simulink library "marlo_lib_v01"  (Simulink 8.1)
settings: Solver=ode45  StartTime=0.0  StopTime=10.0  RelTol=1e-3
undefined symbols (not defined in the file or in its folder): A_deriv_encoder, A_deriv_IMU, ANOMALY_INIT, B_deriv_encoder, B_deriv_IMU, C_deriv_encoder, C_deriv_IMU, CalibrationParams, Com1, D_deriv_encoder, D_deriv_IMU, Dt_deriv_encoder, Dt_deriv_IMU, EncoderAngleLimits, EncoderThreshold, IMUAngleLimits, IMUParams, IMUThreshold, KVHOrientationCal, m_XR17D15x, MAX_ANOMALY, MotorParams, none, standard, x0_deriv_encoder, x0_deriv_IMU, XOFF, XON
libraries: xpcethercatlib x307, speedgoatlib x26, xpcseriallib x15, simulink x8, marlo_lib_v01 x6, dspswit3 x2, xpclib x1
(part 1 of 6)
settings Model: Creator=bgbuss  LastModifiedBy=bgbuss

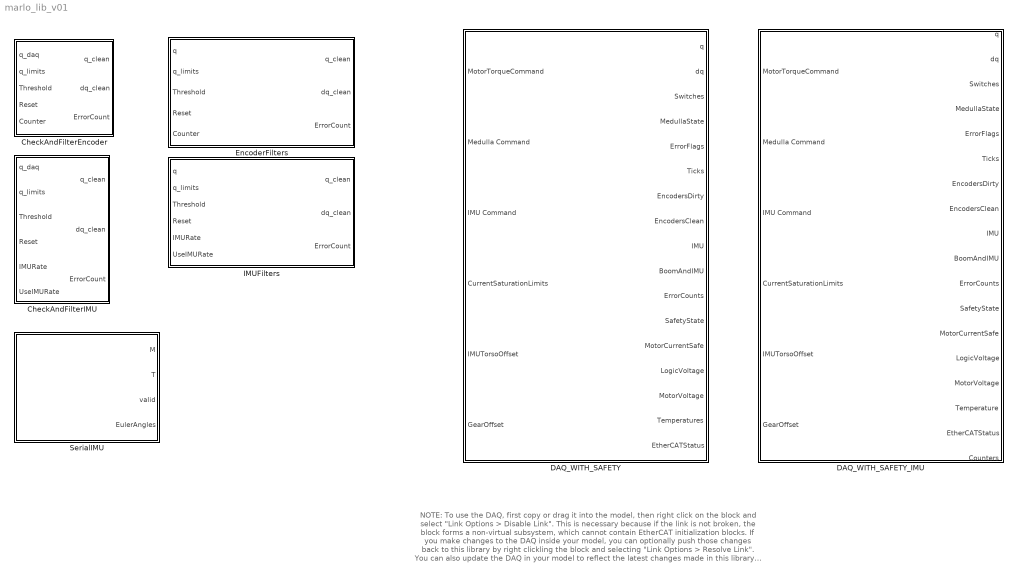
== system marlo_lib_v01 ==
  note: NOTE: To use the DAQ, first copy or drag it into the model,
      | then right click on the block and select "Link Options > Disable Link".
      | This is necessary because if the link is not broken, the block forms a
      | non-virtual subsystem, which cannot contain EtherCAT initialization blocks.
      |
      | If you make changes to the DAQ inside your model, you can optionally push
      | those changes back to this library by right clickling the block and selecting
      | "Link Options > Resolve Link". You can also update the DAQ in your model
      | to reflect the latest changes made in this library by selecting "Link Options >
      | Resolve Link" and pulling (RESTORE) the changes into your model.
  CheckAndFilterEncoder : Subsystem
  CheckAndFilterIMU : Subsystem
  DAQ_WITH_SAFETY : Subsystem
  DAQ_WITH_SAFETY_IMU : Subsystem  AncestorBlock=marlo_lib_v01/DAQ_WITH_SAFETY
  EncoderFilters : Subsystem  TreatAsAtomicUnit=on
  IMUFilters : Subsystem  TreatAsAtomicUnit=on
  SerialIMU : Subsystem

== system marlo_lib_v01/CheckAndFilterEncoder ==
  q_daq : Inport
  q_limits : Inport  Port=2
  Threshold : Inport  Port=3
  Reset : Inport  Port=4
  Counter : Inport  Port=5
  AnomalyDetection : Stateflow chart  TreatAsAtomicUnit=on  SystemSampleTime=Dt_deriv_encoder
  Constant : Constant  Value=Dt_deriv_encoder
  Discrete State-Space : DiscreteStateSpace  A=A_deriv_encoder  B=B_deriv_encoder  C=C_deriv_encoder  D=D_deriv_encoder  X0=x0_deriv_encoder  SampleTime=Dt_deriv_encoder
  Unit Delay : UnitDelay  SampleTime=Dt_deriv_encoder
  q_clean : Outport
  dq_clean : Outport  Port=2
  ErrorCount : Outport  Port=3
  wires:
  AnomalyDetection/1(q_clean) -> Discrete State-Space/1, q_clean/1
  Discrete State-Space/1 -> dq_clean/1, Unit Delay/1
  q_daq/1 -> AnomalyDetection/1(q)
  Threshold/1 -> AnomalyDetection/5(Threshold)
  Unit Delay/1 -> AnomalyDetection/2(dq)
  Constant/1 -> AnomalyDetection/7(ANOMALY_DT)
  q_limits/1 -> AnomalyDetection/4(q_limits)
  AnomalyDetection/2(ErrorCount) -> ErrorCount/1
  Reset/1 -> AnomalyDetection/6(Reset)
  Counter/1 -> AnomalyDetection/3(Counter)

== system marlo_lib_v01/CheckAndFilterIMU ==
  q_daq : Inport
  q_limits : Inport  Port=2
  Threshold : Inport  Port=3
  Reset : Inport  Port=4
  IMURate : Inport  Port=5
  UseIMURate : Inport  Port=6
  AnomalyDetection : Stateflow chart  TreatAsAtomicUnit=on  SystemSampleTime=Dt_deriv_IMU
  Constant : Constant  Value=Dt_deriv_IMU
  Discrete State-Space : DiscreteStateSpace  A=A_deriv_IMU  B=B_deriv_IMU  C=C_deriv_IMU  D=D_deriv_IMU  X0=x0_deriv_IMU  SampleTime=Dt_deriv_IMU
  Rate Transition{,3..7} (6 alike) : RateTransition  OutPortSampleTimeMultiple=2
  Rate Transition1 : RateTransition  Deterministic=off  OutPortSampleTime=.001
  Rate Transition2 : RateTransition  Deterministic=off  OutPortSampleTime=.001
  Rate Transition8 : RateTransition  Deterministic=off  OutPortSampleTime=.001
  Switch : Switch  Criteria=u2 ~= 0  Threshold=0.5
  Unit Delay : UnitDelay  SampleTime=Dt_deriv_IMU
  q_clean : Outport
  dq_clean : Outport  Port=2
  ErrorCount : Outport  Port=3
  wires:
  Unit Delay/1 -> AnomalyDetection/2(dq)
  Threshold/1 -> Rate Transition5/1
  q_daq/1 -> Rate Transition/1
  AnomalyDetection/1(q_clean) -> Discrete State-Space/1, Rate Transition1/1
  Rate Transition/1 -> AnomalyDetection/1(q)
  Rate Transition1/1 -> q_clean/1
  Rate Transition2/1 -> dq_clean/1
  Switch/1 -> Rate Transition2/1, Unit Delay/1
  Discrete State-Space/1 -> Switch/3
  IMURate/1 -> Rate Transition3/1
  UseIMURate/1 -> Rate Transition4/1
  Constant/1 -> AnomalyDetection/6(ANOMALY_DT)
  Rate Transition3/1 -> Switch/1
  Rate Transition4/1 -> Switch/2
  Rate Transition5/1 -> AnomalyDetection/4(Threshold)
  q_limits/1 -> Rate Transition6/1
  Reset/1 -> Rate Transition7/1
  Rate Transition6/1 -> AnomalyDetection/3(q_limits)
  Rate Transition7/1 -> AnomalyDetection/5(Reset)
  AnomalyDetection/2(ErrorCount) -> Rate Transition8/1
  Rate Transition8/1 -> ErrorCount/1

== system marlo_lib_v01/DAQ_WITH_SAFETY ==
  MotorTorqueCommand : Inport
  Medulla Command : Inport  Port=2
  IMU Command : Inport  Port=3
  CurrentSaturationLimits : Inport  Port=4
  IMUTorsoOffset : Inport  Port=5
  GearOffset : Inport  Port=6
  DAQ : Subsystem
  Data Type Conversion15 : DataTypeConversion  OutDataTypeStr=double
  Gain : Gain  Gain=-1
  SAFETY : MATLAB Function  TreatAsAtomicUnit=on
  Saturation Dynamic : simulink/Discontinuities/Saturation Dynamic  OutMin=[]  OutMax=[]  OutDataTypeStr=Inherit: Same as second input  OutDataType=fixdt(1, 16)  OutScaling=2^-10  DoSatur=off
  Terminator2 : Terminator
  Terminator5 : Terminator
  TorqueToCurrent : Gain  Gain=[10; 10; 5.5; 10; 10; 5.5]
  Unit Delay : UnitDelay  SampleTime=-1
  q : Outport
  dq : Outport  Port=2
  Switches : Outport  Port=3
  MedullaState : Outport  Port=4
  ErrorFlags : Outport  Port=5
  Ticks : Outport  Port=6
  EncodersDirty : Outport  Port=7
  EncodersClean : Outport  Port=8
  IMU : Outport  Port=9
  BoomAndIMU : Outport  Port=10
  ErrorCounts : Outport  Port=11
  SafetyState : Outport  Port=12
  MotorCurrentSafe : Outport  Port=13
  LogicVoltage : Outport  Port=14
  MotorVoltage : Outport  Port=15
  Temperatures : Outport  Port=16
  EtherCATStatus : Outport  Port=17
  wires:
  DAQ/17(EtherCATStatus) -> EtherCATStatus/1
  DAQ/4(ToeSwitches) -> Terminator2/1
  DAQ/12(EncodersDirty) -> EncodersDirty/1
  DAQ/11(Ticks) -> Ticks/1
  SAFETY/3(IMUCommandSafe) -> DAQ/3(IMU Command)
  MotorTorqueCommand/1 -> TorqueToCurrent/1
  Medulla Command/1 -> SAFETY/2(MedullaCommand)
  IMU Command/1 -> SAFETY/3(IMUCommand)
  DAQ/1(q) -> SAFETY/4(q), q/1
  DAQ/2(dq) -> SAFETY/5(dq), dq/1
  DAQ/3(LimitSwitches) -> SAFETY/6(Switches), Switches/1
  DAQ/8(LogicVoltage) -> LogicVoltage/1, SAFETY/8(LogicVoltage)
  DAQ/14(IMU) -> IMU/1
  SAFETY/4(SafetyStateOut) -> SafetyState/1
  TorqueToCurrent/1 -> Saturation Dynamic/2  "current_unsat"
  DAQ/10(Thermistors) -> Temperatures/1, SAFETY/7(Thermistors)
  DAQ/7(MotorVoltage) -> MotorVoltage/1
  DAQ/9(AmpMeasuredCurrent) -> Terminator5/1
  DAQ/5(MedullaState) -> MedullaState/1
  DAQ/6(ErrorFlags) -> ErrorFlags/1
  Saturation Dynamic/1 -> Data Type Conversion15/1
  CurrentSaturationLimits/1 -> Saturation Dynamic/1, Gain/1
  Gain/1 -> Saturation Dynamic/3
  SAFETY/1(MotorCurrentCommandSafe) -> DAQ/1(Motor Command), MotorCurrentSafe/1
  SAFETY/2(MedullaCommandSafe) -> DAQ/2(Medulla Command)
  Data Type Conversion15/1 -> SAFETY/1(MotorCurrentCommand)  "current_sat"
  DAQ/15(BoomAndIMU) -> BoomAndIMU/1
  IMUTorsoOffset/1 -> DAQ/4(IMUTorsoOffset)
  GearOffset/1 -> DAQ/5(GearOffset)
  SAFETY/5(SafetyCountOut) -> Unit Delay/1
  Unit Delay/1 -> SAFETY/9(SafetyCountIn)
  DAQ/16(ErrorCounts) -> ErrorCounts/1
  DAQ/13(EncodersClean) -> EncodersClean/1

== system marlo_lib_v01/DAQ_WITH_SAFETY_IMU ==
  MotorTorqueCommand : Inport
  Medulla Command : Inport  Port=2
  IMU Command : Inport  Port=3
  CurrentSaturationLimits : Inport  Port=4
  IMUTorsoOffset : Inport  Port=5
  GearOffset : Inport  Port=6
  DAQ : Subsystem
  Data Type Conversion15 : DataTypeConversion  OutDataTypeStr=double
  Gain : Gain  Gain=-1
  SAFETY : MATLAB Function  TreatAsAtomicUnit=on
  Saturation Dynamic : simulink/Discontinuities/Saturation Dynamic  OutMin=[]  OutMax=[]  OutDataTypeStr=Inherit: Same as second input  OutDataType=fixdt(1, 16)  OutScaling=2^-10  DoSatur=off
  Terminator2 : Terminator
  Terminator5 : Terminator
  TorqueToCurrent : Gain  Gain=[10; 10; 5.5; 10; 10; 5.5]
  Unit Delay : UnitDelay  SampleTime=-1
  q : Outport
  dq : Outport  Port=2
  Switches : Outport  Port=3
  MedullaState : Outport  Port=4
  ErrorFlags : Outport  Port=5
  Ticks : Outport  Port=6
  EncodersDirty : Outport  Port=7
  EncodersClean : Outport  Port=8
  IMU : Outport  Port=9
  BoomAndIMU : Outport  Port=10
  ErrorCounts : Outport  Port=11
  SafetyState : Outport  Port=12
  MotorCurrentSafe : Outport  Port=13
  LogicVoltage : Outport  Port=14
  MotorVoltage : Outport  Port=15
  Temperature : Outport  Port=16
  EtherCATStatus : Outport  Port=17
  Counters : Outport  Port=18
  wires:
  DAQ/19(Counters) -> Counters/1
  DAQ/18(TemperatureMuxed) -> Temperature/1
  DAQ/13(EncodersClean) -> EncodersClean/1
  DAQ/16(ErrorCounts) -> ErrorCounts/1
  Unit Delay/1 -> SAFETY/9(SafetyCountIn)
  SAFETY/5(SafetyCountOut) -> Unit Delay/1
  GearOffset/1 -> DAQ/5(GearOffset)
  IMUTorsoOffset/1 -> DAQ/4(IMUTorsoOffset)
  DAQ/15(BoomAndIMU) -> BoomAndIMU/1
  Data Type Conversion15/1 -> SAFETY/1(MotorCurrentCommand)  "current_sat"
  SAFETY/2(MedullaCommandSafe) -> DAQ/2(Medulla Command)
  SAFETY/1(MotorCurrentCommandSafe) -> DAQ/1(Motor Command), MotorCurrentSafe/1
  Gain/1 -> Saturation Dynamic/3
  CurrentSaturationLimits/1 -> Gain/1, Saturation Dynamic/1
  Saturation Dynamic/1 -> Data Type Conversion15/1
  DAQ/6(ErrorFlags) -> ErrorFlags/1
  DAQ/5(MedullaState) -> MedullaState/1
  DAQ/9(AmpMeasuredCurrent) -> Terminator5/1
  DAQ/7(MotorVoltage) -> MotorVoltage/1
  DAQ/10(Thermistors) -> SAFETY/7(Thermistors)
  TorqueToCurrent/1 -> Saturation Dynamic/2  "current_unsat"
  SAFETY/4(SafetyStateOut) -> SafetyState/1
  DAQ/14(IMU) -> IMU/1
  DAQ/8(LogicVoltage) -> LogicVoltage/1, SAFETY/8(LogicVoltage)
  DAQ/3(LimitSwitches) -> Switches/1, SAFETY/6(Switches)
  DAQ/2(dq) -> dq/1, SAFETY/5(dq)
  DAQ/1(q) -> q/1, SAFETY/4(q)
  IMU Command/1 -> SAFETY/3(IMUCommand)
  Medulla Command/1 -> SAFETY/2(MedullaCommand)
  MotorTorqueCommand/1 -> TorqueToCurrent/1
  SAFETY/3(IMUCommandSafe) -> DAQ/3(IMU Command)
  DAQ/11(Ticks) -> Ticks/1
  DAQ/12(EncodersDirty) -> EncodersDirty/1
  DAQ/4(ToeSwitches) -> Terminator2/1
  DAQ/17(EtherCATStatus) -> EtherCATStatus/1

== system marlo_lib_v01/EncoderFilters ==
  q : Inport  Partition=on  PartitionDimension=1  PartitionWidth=1
  q_limits : Inport  Port=2  Partition=on  PartitionDimension=1  PartitionWidth=1
  Threshold : Inport  Port=3  Partition=on  PartitionDimension=1  PartitionWidth=1
  Reset : Inport  Port=4  Partition=off
  Counter : Inport  Port=5  Partition=on  PartitionDimension=1  PartitionWidth=1
  CheckAndFilterEncoder : marlo_lib_v01/CheckAndFilterEncoder
  For Each : ForEach  DisableCoverage=on  IndexMode=One-based
  q_clean : Outport  ConcatenationDimension=1
  dq_clean : Outport  Port=2  ConcatenationDimension=1
  ErrorCount : Outport  Port=3  ConcatenationDimension=1
  wires:
  q/1 -> CheckAndFilterEncoder/1
  Threshold/1 -> CheckAndFilterEncoder/3
  CheckAndFilterEncoder/1 -> q_clean/1
  CheckAndFilterEncoder/3 -> ErrorCount/1
  q_limits/1 -> CheckAndFilterEncoder/2
  CheckAndFilterEncoder/2 -> dq_clean/1
  Reset/1 -> CheckAndFilterEncoder/4
  Counter/1 -> CheckAndFilterEncoder/5

== system marlo_lib_v01/IMUFilters ==
  q : Inport  Partition=on  PartitionDimension=1  PartitionWidth=1
  q_limits : Inport  Port=2  Partition=on  PartitionDimension=1  PartitionWidth=1
  Threshold : Inport  Port=3  Partition=off
  Reset : Inport  Port=4  Partition=off
  IMURate : Inport  Port=5  Partition=on  PartitionDimension=1  PartitionWidth=1
  UseIMURate : Inport  Port=6  Partition=off
  CheckAndFilterIMU : marlo_lib_v01/CheckAndFilterIMU
  For Each : ForEach  DisableCoverage=on  IndexMode=One-based
  q_clean : Outport  ConcatenationDimension=1
  dq_clean : Outport  Port=2  ConcatenationDimension=1
  ErrorCount : Outport  Port=3  ConcatenationDimension=1
  wires:
  Reset/1 -> CheckAndFilterIMU/4
  CheckAndFilterIMU/2 -> dq_clean/1
  q_limits/1 -> CheckAndFilterIMU/2
  CheckAndFilterIMU/3 -> ErrorCount/1
  CheckAndFilterIMU/1 -> q_clean/1
  Threshold/1 -> CheckAndFilterIMU/3
  q/1 -> CheckAndFilterIMU/1
  IMURate/1 -> CheckAndFilterIMU/5
  UseIMURate/1 -> CheckAndFilterIMU/6

== system marlo_lib_v01/SerialIMU ==
  Baseboard Serial F : xpcseriallib/Mainboard/Baseboard Serial F  group=Basic Setup  port=1  irqnum=4  saddr1=0x3f8  saddr2=0x3e8  config=Com1/none  baud1=115200  parity1=None  ndata1=8  nstop1=1  fifomode1=16 deep  rlevel1=1  automode1=off  xmtfifosize1=1024  xmtdatatype1=8 bit uint null terminated  rcvfifosize1=1024  baud2=115200  parity2=None  ndata2=8  nstop2=1  fifomode2=16 deep  rlevel2=half full  automode2=off  xmtfifosize2=1024  xmtdatatype2=8 bit uint null terminated  rcvfifosize2=1024
  Constant : Constant  Value=IMUParams
  "FIFO bin read " : xpcseriallib/FIFO bin read   header={char(hex2dec('c5'))}  lengths=[43]  hold=Zero output if no new data  enable=off  maxsize=64  outputtype=8 bit uint null terminated  sampletime=0.001
  Ground : Ground
  Ground1 : Ground
  MATLAB Function : MATLAB Function  TreatAsAtomicUnit=on
  M_to_Euler : MATLAB Function  TreatAsAtomicUnit=on
  Reshape : Reshape  OutputDimensionality=Customize  OutputDimensions=[3,3]
  Terminator2 : Terminator
  M : Outport  PortDimensions=9
  T : Outport  Port=2
  valid : Outport  Port=3
  EulerAngles : Outport  Port=4
  wires:
  Ground/1 -> Baseboard Serial F/2
  Ground1/1 -> Baseboard Serial F/1
  Baseboard Serial F/1 -> "FIFO bin read "/1
  Baseboard Serial F/2 -> Terminator2/1
  "FIFO bin read "/1 -> MATLAB Function/1(D)
  MATLAB Function/1(M) -> Reshape/1, M/1
  MATLAB Function/2(T) -> T/1
  MATLAB Function/3(valid) -> valid/1
  M_to_Euler/1(EulerAngles) -> EulerAngles/1
  Reshape/1 -> M_to_Euler/1(M_WI)
  Constant/1 -> M_to_Euler/2(IMUParams)

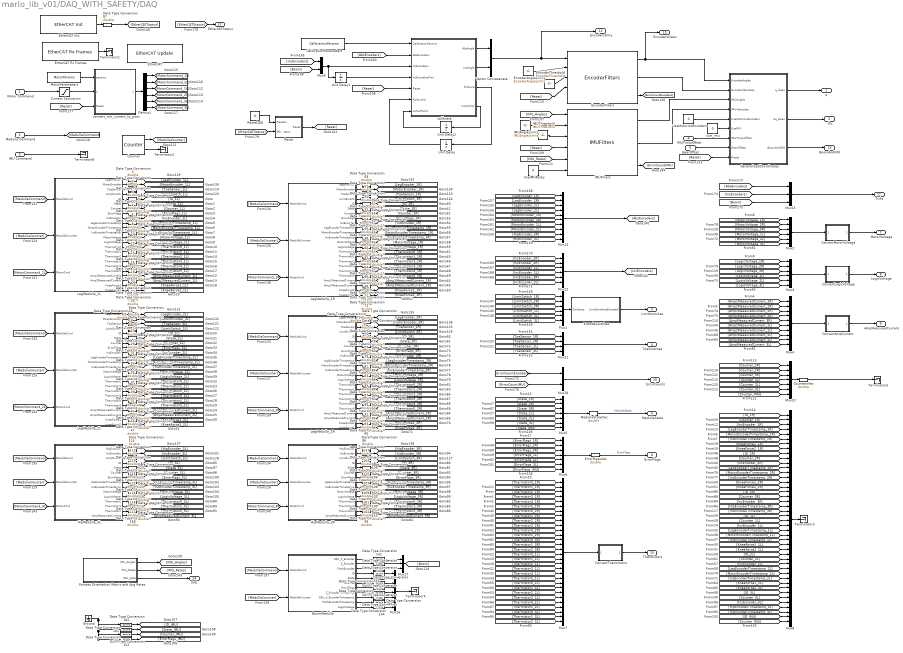
== system marlo_lib_v01/DAQ_WITH_SAFETY/DAQ ==
  Motor Command : Inport
  Medulla Command : Inport  Port=2
  IMU Command : Inport  Port=3
  IMUTorsoOffset : Inport  Port=4
  GearOffset : Inport  Port=5
  BoomMedulla : Subsystem
  CalibrationParameters : Constant  Value=CalibrationParams
  ConvertAmpCurrent : MATLAB Function  TreatAsAtomicUnit=on
  ConvertLogicVoltage : MATLAB Function  TreatAsAtomicUnit=on
  ConvertMotorVoltage : MATLAB Function  TreatAsAtomicUnit=on
  ConvertThermistors : MATLAB Function  TreatAsAtomicUnit=on
  Counter : dspswit3/Counter  Direction=Up  CountEvent=Free running  CounterSize=User defined  MaxCount=65535  InitialCount=0  Output=Count and Hit  HitValue=32  ResetInput=off  SamplesPerFrame=1  Ts=.001  CntDtype=double  HitDtype=Logical
  CountersVec : DataTypeConversion  OutDataTypeStr=double
  Current Saturation : Saturate  UpperLimit=50  LowerLimit=-50
  Data Type Conversion{1..112,114..126,131..133,138..145,152,154,157..158,161..162} (142 alike) : DataTypeConversion  OutDataTypeStr=double
  Demux1 : Demux  Outputs=6
  EncodeSwitches : MATLAB Function  TreatAsAtomicUnit=on
  EncoderAngleLimits : Constant  Value=EncoderAngleLimits
  EncoderFilters : marlo_lib_v01/EncoderFilters
  EncoderThreshold : Constant  Value=EncoderThreshold
  ErrorFlagsVec : DataTypeConversion  OutDataTypeStr=double
  EtherCAT : xpcethercatlib/EtherCAT Update   Priority=4  device_id=0  task_id_list=[1]  task_rates=[1]  task_priorities=[1500]
  EtherCAT Init : xpcethercatlib/EtherCAT Init   Priority=0  config_file='full_robot_eni_v4.xml'  device_id=0  pci_bus=5  pci_slot=5  enaDC=on  errRptLevel=0  sample_time=-1
  EtherCAT Rx Frames : xpcethercatlib/EtherCAT Rx Frames   Priority=1  device_id=0  sample_time=0
  GeneralizedCoordinates : MATLAB Function  TreatAsAtomicUnit=on
  Ground : Ground
  HipMedulla_3L : Subsystem
  HipMedulla_3R : Subsystem
  IMUAngleLimits : Constant  Value=IMUAngleLimits
  IMUFilters : marlo_lib_v01/IMUFilters
  IMUThreshold : Constant  Value=IMUThreshold
  LegMedulla_1L : Subsystem
  LegMedulla_1R : Subsystem
  LegMedulla_2L : Subsystem
  LegMedulla_2R : Subsystem
  MedullaStateVec : DataTypeConversion  OutDataTypeStr=double
  MotorParameters : Constant  Value=MotorParams
  Mux{1..3,12} (4 alike) : Mux  Inputs=6
  Mux10 : Mux  Inputs=7
  Mux11 : Mux
  Mux14 : Mux  Inputs=10
  Mux15 : Mux  Inputs=3
  Mux16 : Mux  Inputs=8
  Mux17 : Mux  Inputs=3
  Mux18 : Mux  Inputs=2
  Mux4 : Mux  Inputs=10
  Mux5 : Mux  Inputs=7
  Mux6 : Mux  Inputs=7
  Mux7 : Mux  Inputs=30
  Mux8 : Mux  Inputs=44
  Mux9 : Mux  Inputs=2
  Process Orientation Matrix and Ang Rates : Subsystem
  Reset : Subsystem
  ResetDAQ : Constant  Value=0
  Terminator{1..5,8} (6 alike) : Terminator
  Unit Delay : UnitDelay  InitialCondition=zeros(9,1)  SampleTime=-1
  Unit Delay1 : UnitDelay  SampleTime=-1
  Unit Delay2 : UnitDelay  InitialCondition=zeros(6,1)  SampleTime=-1
  UseIMURates : Constant  Value=0
  UseMotorIncEncoders : Constant  Value=0
  Vector Concatenate : Concatenate
  calibrate : MATLAB Function  TreatAsAtomicUnit=on
  convert_mtr_current_to_pwm : MATLAB Function  TreatAsAtomicUnit=on
  use_imu : Constant  Value=0
  q : Outport
  dq : Outport  Port=2
  LimitSwitches : Outport  Port=3
  ToeSwitches : Outport  Port=4
  MedullaState : Outport  Port=5
  ErrorFlags : Outport  Port=6
  MotorVoltage : Outport  Port=7
  LogicVoltage : Outport  Port=8
  AmpMeasuredCurrent : Outport  Port=9
  Thermistors : Outport  Port=10
  Ticks : Outport  Port=11
  EncodersDirty : Outport  Port=12
  EncodersClean : Outport  Port=13
  IMU : Outport  Port=14
  BoomAndIMU : Outport  Port=15
  ErrorCounts : Outport  Port=16
  EtherCATStatus : Outport  Port=17
  wires:
  [EtherCATStatus] -> Reset/2(EtherCATStatus)
  [EtherCATStatus] -> EtherCATStatus/1
  Data Type Conversion97/1 -> [EtherCATStatus]
  [Reset] -> convert_mtr_current_to_pwm/3(Reset)
  BoomMedulla/1(OSU_X_Encoder) -> Data Type Conversion141/1
  BoomMedulla/2(Z_Encoder) -> Data Type Conversion140/1
  EtherCAT Init/1 -> Data Type Conversion97/1
  Mux11/1 -> ToeSwitches/1
  EncodeSwitches/1(LimitSwitchesEncoded) -> LimitSwitches/1
  LegMedulla_1L/2(MotorEncoder) -> Data Type Conversion1/1
  LegMedulla_1L/3(ToeSensor) -> Data Type Conversion2/1
  LegMedulla_1L/4(LimitSwitch) -> Data Type Conversion4/1
  LegMedulla_1L/5(ID) -> Data Type Conversion5/1
  LegMedulla_1L/6(State) -> Data Type Conversion6/1
  LegMedulla_1L/7(Counter) -> Data Type Conversion7/1
  LegMedulla_1L/8(ErrorFlags) -> Data Type Conversion8/1
  LegMedulla_1L/9(IncEncoder) -> Data Type Conversion9/1
  LegMedulla_1L/10(LegEncoderTimestamp) -> Data Type Conversion10/1
  LegMedulla_1L/11(MotorEncoderTimestamp) -> Data Type Conversion11/1
  LegMedulla_1L/12(IncEncoderTimestamp) -> Data Type Conversion12/1
  LegMedulla_1L/13(MotorVoltage) -> Data Type Conversion13/1
  LegMedulla_1L/14(LogicVoltage) -> Data Type Conversion14/1
  LegMedulla_1L/15(Thermistor0) -> Data Type Conversion15/1
  LegMedulla_1L/16(Thermistor1) -> Data Type Conversion16/1
  LegMedulla_1L/17(Thermistor2) -> Data Type Conversion17/1
  LegMedulla_1L/18(Thermistor3) -> Data Type Conversion18/1
  LegMedulla_1L/19(Thermistor4) -> Data Type Conversion19/1
  LegMedulla_1L/20(Thermistor5) -> Data Type Conversion20/1
  LegMedulla_1L/21(Amp1MeasuredCurrent) -> Data Type Conversion21/1
  LegMedulla_1L/22(Amp2MeasuredCurrent) -> Data Type Conversion22/1
  LegMedulla_1L/23(KneeForce1) -> Data Type Conversion23/1
  LegMedulla_2L/1(LegEncoder) -> Data Type Conversion25/1
  LegMedulla_2L/2(MotorEncoder) -> Data Type Conversion26/1
  LegMedulla_2L/3(ToeSensor) -> Data Type Conversion27/1
  LegMedulla_2L/4(LimitSwitch) -> Data Type Conversion28/1
  LegMedulla_2L/5(ID) -> Data Type Conversion29/1
  LegMedulla_2L/6(State) -> Data Type Conversion30/1
  LegMedulla_2L/7(Counter) -> Data Type Conversion31/1
  LegMedulla_2L/8(ErrorFlags) -> Data Type Conversion32/1
  LegMedulla_2L/9(IncEncoder) -> Data Type Conversion33/1
  LegMedulla_2L/10(LegEncoderTimestamp) -> Data Type Conversion34/1
  LegMedulla_2L/11(MotorEncoderTimestamp) -> Data Type Conversion35/1
  LegMedulla_2L/12(IncEncoderTimestamp) -> Data Type Conversion36/1
  LegMedulla_2L/13(MotorVoltage) -> Data Type Conversion37/1
  LegMedulla_2L/14(LogicVoltage) -> Data Type Conversion38/1
  LegMedulla_2L/15(Thermistor0) -> Data Type Conversion39/1
  LegMedulla_2L/16(Thermistor1) -> Data Type Conversion40/1
  LegMedulla_2L/17(Thermistor2) -> Data Type Conversion41/1
  LegMedulla_2L/18(Thermistor3) -> Data Type Conversion42/1
  LegMedulla_2L/19(Thermistor4) -> Data Type Conversion43/1
  LegMedulla_2L/20(Thermistor5) -> Data Type Conversion44/1
  LegMedulla_2L/21(Amp1MeasuredCurrent) -> Data Type Conversion45/1
  LegMedulla_2L/22(Amp2MeasuredCurrent) -> Data Type Conversion46/1
  LegMedulla_2L/23(KneeForce1) -> Data Type Conversion47/1
  LegMedulla_1L/24(KneeForce2) -> Data Type Conversion24/1
  LegMedulla_2L/24(KneeForce2) -> Data Type Conversion48/1
  LegMedulla_1R/3(ToeSensor) -> Data Type Conversion51/1
  LegMedulla_1R/4(LimitSwitch) -> Data Type Conversion52/1
  LegMedulla_1R/5(ID) -> Data Type Conversion53/1
  LegMedulla_1R/6(State) -> Data Type Conversion54/1
  LegMedulla_1R/7(Counter) -> Data Type Conversion55/1
  LegMedulla_1R/8(ErrorFlags) -> Data Type Conversion56/1
  LegMedulla_1R/9(IncEncoder) -> Data Type Conversion57/1
  LegMedulla_1R/10(LegEncoderTimestamp) -> Data Type Conversion58/1
  LegMedulla_1R/11(MotorEncoderTimestamp) -> Data Type Conversion59/1
  LegMedulla_1R/12(IncEncoderTimestamp) -> Data Type Conversion60/1
  LegMedulla_1R/13(MotorVoltage) -> Data Type Conversion61/1
  LegMedulla_1R/14(LogicVoltage) -> Data Type Conversion62/1
  LegMedulla_1R/15(Thermistor0) -> Data Type Conversion63/1
  LegMedulla_1R/16(Thermistor1) -> Data Type Conversion64/1
  LegMedulla_1R/17(Thermistor2) -> Data Type Conversion65/1
  LegMedulla_1R/18(Thermistor3) -> Data Type Conversion66/1
  LegMedulla_1R/19(Thermistor4) -> Data Type Conversion67/1
  LegMedulla_1R/20(Thermistor5) -> Data Type Conversion68/1
  LegMedulla_1R/21(Amp1MeasuredCurrent) -> Data Type Conversion69/1
  LegMedulla_1R/22(Amp2MeasuredCurrent) -> Data Type Conversion70/1
  LegMedulla_1R/23(KneeForce1) -> Data Type Conversion71/1
  LegMedulla_2R/4(LimitSwitch) -> Data Type Conversion76/1
  LegMedulla_2R/5(ID) -> Data Type Conversion77/1
  LegMedulla_2R/6(State) -> Data Type Conversion78/1
  LegMedulla_2R/7(Counter) -> Data Type Conversion79/1
  LegMedulla_2R/8(ErrorFlags) -> Data Type Conversion80/1
  LegMedulla_2R/9(IncEncoder) -> Data Type Conversion81/1
  LegMedulla_2R/10(LegEncoderTimestamp) -> Data Type Conversion82/1
  LegMedulla_2R/11(MotorEncoderTimestamp) -> Data Type Conversion83/1
  LegMedulla_2R/12(IncEncoderTimestamp) -> Data Type Conversion84/1
  LegMedulla_2R/13(MotorVoltage) -> Data Type Conversion85/1
  LegMedulla_2R/14(LogicVoltage) -> Data Type Conversion86/1
  LegMedulla_2R/15(Thermistor0) -> Data Type Conversion87/1
  LegMedulla_2R/16(Thermistor1) -> Data Type Conversion88/1
  LegMedulla_2R/17(Thermistor2) -> Data Type Conversion89/1
  LegMedulla_2R/18(Thermistor3) -> Data Type Conversion90/1
  LegMedulla_2R/19(Thermistor4) -> Data Type Conversion91/1
  LegMedulla_2R/20(Thermistor5) -> Data Type Conversion92/1
  LegMedulla_2R/21(Amp1MeasuredCurrent) -> Data Type Conversion93/1
  LegMedulla_2R/22(Amp2MeasuredCurrent) -> Data Type Conversion94/1
  LegMedulla_2R/23(KneeForce1) -> Data Type Conversion95/1
  LegMedulla_1R/24(KneeForce2) -> Data Type Conversion72/1
  LegMedulla_2R/24(KneeForce2) -> Data Type Conversion96/1
  Medulla Command/1 -> [MedullaCommand]
  EtherCAT Rx Frames/1 -> Terminator1/1
  Counter/2 -> Terminator2/1
  LegMedulla_2R/1(LegEncoder) -> Data Type Conversion73/1
  LegMedulla_2R/2(MotorEncoder) -> Data Type Conversion74/1
  LegMedulla_2R/3(ToeSensor) -> Data Type Conversion75/1
  Data Type Conversion53/1 -> [ID_1R]
  Data Type Conversion54/1 -> [State_1R]
  Data Type Conversion55/1 -> [Counter_1R]
  Data Type Conversion56/1 -> [ErrorFlags_1R]
  Data Type Conversion57/1 -> [IncEncoder_1R]
  Data Type Conversion58/1 -> [LegEncoderTimestamp_1R]
  Data Type Conversion59/1 -> [MotorEncoderTimestamp_1R]
  Data Type Conversion60/1 -> [IncEncoderTimestamp_1R]
  Data Type Conversion61/1 -> [MotorVoltage_1R]
  Data Type Conversion62/1 -> [LogicVoltage_1R]
  Data Type Conversion63/1 -> [Thermistor0_1R]
  Data Type Conversion64/1 -> [Thermistor1_1R]
  Data Type Conversion65/1 -> [Thermistor2_1R]
  Data Type Conversion66/1 -> [Thermistor3_1R]
  Data Type Conversion67/1 -> [Thermistor4_1R]
  Data Type Conversion68/1 -> [Thermistor5_1R]
  Data Type Conversion69/1 -> [Amp1MeasuredCurrent_1R]
  Data Type Conversion70/1 -> [Amp2MeasuredCurrent_1R]
  Data Type Conversion71/1 -> [KneeForce1_1R]
  Data Type Conversion72/1 -> [KneeForce2_1R]
  Data Type Conversion77/1 -> [ID_2R]
  Data Type Conversion78/1 -> [State_2R]
  Data Type Conversion79/1 -> [Counter_2R]
  Data Type Conversion80/1 -> [ErrorFlags_2R]
  Data Type Conversion81/1 -> [IncEncoder_2R]
  Data Type Conversion82/1 -> [LegEncoderTimestamp_2R]
  Data Type Conversion83/1 -> [MotorEncoderTimestamp_2R]
  Data Type Conversion84/1 -> [IncEncoderTimestamp_2R]
  Data Type Conversion85/1 -> [MotorVoltage_2R]
  Data Type Conversion86/1 -> [LogicVoltage_2R]
  Data Type Conversion87/1 -> [Thermistor0_2R]
  Data Type Conversion88/1 -> [Thermistor1_2R]
  Data Type Conversion89/1 -> [Thermistor2_2R]
  Data Type Conversion90/1 -> [Thermistor3_2R]
  Data Type Conversion91/1 -> [Thermistor4_2R]
  Data Type Conversion92/1 -> [Thermistor5_2R]
  Data Type Conversion93/1 -> [Amp1MeasuredCurrent_2R]
  Data Type Conversion94/1 -> [Amp2MeasuredCurrent_2R]
  Data Type Conversion95/1 -> [KneeForce1_2R]
  Data Type Conversion96/1 -> [KneeForce2_2R]
  Data Type Conversion111/1 -> [AmpMeasuredCurrent_3R]
  Motor Command/1 -> Current Saturation/1
  MotorParameters/1 -> convert_mtr_current_to_pwm/1(params)
  Current Saturation/1 -> convert_mtr_current_to_pwm/2(u)
  LegMedulla_1R/2(MotorEncoder) -> Data Type Conversion50/1
  LegMedulla_1L/1(LegEncoder) -> Data Type Conversion3/1
  LegMedulla_1R/1(LegEncoder) -> Data Type Conversion49/1
  Data Type Conversion5/1 -> [ID_1L]
  Data Type Conversion6/1 -> [State_1L]
  Data Type Conversion7/1 -> [Counter_1L]
  Data Type Conversion29/1 -> [ID_2L]
  Data Type Conversion30/1 -> [State_2L]
  Data Type Conversion31/1 -> [Counter_2L]
  Data Type Conversion32/1 -> [ErrorFlags_2L]
  Data Type Conversion33/1 -> [IncEncoder_2L]
  Data Type Conversion34/1 -> [LegEncoderTimestamp_2L]
  Data Type Conversion35/1 -> [MotorEncoderTimestamp_2L]
  Data Type Conversion36/1 -> [IncEncoderTimestamp_2L]
  Data Type Conversion37/1 -> [MotorVoltage_2L]
  Data Type Conversion38/1 -> [LogicVoltage_2L]
  Data Type Conversion39/1 -> [Thermistor0_2L]
  Data Type Conversion40/1 -> [Thermistor1_2L]
  Data Type Conversion41/1 -> [Thermistor2_2L]
  Data Type Conversion42/1 -> [Thermistor3_2L]
  Data Type Conversion43/1 -> [Thermistor4_2L]
  Data Type Conversion44/1 -> [Thermistor5_2L]
  Data Type Conversion45/1 -> [Amp1MeasuredCurrent_2L]
  Data Type Conversion46/1 -> [Amp2MeasuredCurrent_2L]
  Data Type Conversion47/1 -> [KneeForce1_2L]
  Data Type Conversion48/1 -> [KneeForce2_2L]
  convert_mtr_current_to_pwm/1(y) -> Demux1/1
  Data Type Conversion99/1 -> [Thermistor2_3R]
  Data Type Conversion100/1 -> [Thermistor1_3R]
  Data Type Conversion102/1 -> [Thermistor0_3R]
  Data Type Conversion103/1 -> [LogicVoltage_3R]
  Data Type Conversion101/1 -> [MotorVoltage_3R]
  Data Type Conversion108/1 -> [IncEncoderTimestamp_3R]
  Data Type Conversion109/1 -> [HipEncoderTimestamp_3R]
  Data Type Conversion104/1 -> [IncEncoder_3R]
  Data Type Conversion106/1 -> [ErrorFlags_3R]
  Data Type Conversion107/1 -> [Counter_3R]
  Data Type Conversion105/1 -> [State_3R]
  Data Type Conversion110/1 -> [ID_3R]
  Data Type Conversion98/1 -> [HipEncoder_3R]
  HipMedulla_3R/1(HipEncoder) -> Data Type Conversion98/1
  HipMedulla_3R/2(IncEncoder) -> Data Type Conversion104/1
  HipMedulla_3R/3(LimitSwitch) -> Data Type Conversion157/1
  HipMedulla_3R/4(ID) -> Data Type Conversion110/1
  HipMedulla_3R/5(State) -> Data Type Conversion105/1
  HipMedulla_3R/6(Counter) -> Data Type Conversion107/1
  HipMedulla_3R/7(ErrorFlags) -> Data Type Conversion106/1
  HipMedulla_3R/8(HipEncoderTimestamp) -> Data Type Conversion109/1
  HipMedulla_3R/9(IncEncoderTimestamp) -> Data Type Conversion108/1
  HipMedulla_3R/10(MotorVoltage) -> Data Type Conversion101/1
  HipMedulla_3R/11(LogicVoltage) -> Data Type Conversion103/1
  HipMedulla_3R/12(Thermistor0) -> Data Type Conversion102/1
  HipMedulla_3R/13(Thermistor1) -> Data Type Conversion100/1
  HipMedulla_3R/14(Thermistor2) -> Data Type Conversion99/1
  HipMedulla_3R/15(AmpMeasuredCurrent) -> Data Type Conversion111/1
  HipMedulla_3L/3(LimitSwitch) -> Data Type Conversion112/1
  Data Type Conversion114/1 -> [HipEncoder_3L]
  HipMedulla_3L/1(HipEncoder) -> Data Type Conversion114/1
  HipMedulla_3L/2(IncEncoder) -> Data Type Conversion119/1
  Data Type Conversion126/1 -> [AmpMeasuredCurrent_3L]
  Data Type Conversion158/1 -> [Thermistor2_3L]
  Data Type Conversion115/1 -> [Thermistor1_3L]
  Data Type Conversion117/1 -> [Thermistor0_3L]
  Data Type Conversion118/1 -> [LogicVoltage_3L]
  Data Type Conversion116/1 -> [MotorVoltage_3L]
  Data Type Conversion123/1 -> [IncEncoderTimestamp_3L]
  Data Type Conversion124/1 -> [HipEncoderTimestamp_3L]
  Data Type Conversion119/1 -> [IncEncoder_3L]
  Data Type Conversion121/1 -> [ErrorFlags_3L]
  Data Type Conversion122/1 -> [Counter_3L]
  Data Type Conversion120/1 -> [State_3L]
  Data Type Conversion125/1 -> [ID_3L]
  HipMedulla_3L/4(ID) -> Data Type Conversion125/1
  HipMedulla_3L/5(State) -> Data Type Conversion120/1
  HipMedulla_3L/6(Counter) -> Data Type Conversion122/1
  HipMedulla_3L/7(ErrorFlags) -> Data Type Conversion121/1
  HipMedulla_3L/8(HipEncoderTimestamp) -> Data Type Conversion124/1
  HipMedulla_3L/9(IncEncoderTimestamp) -> Data Type Conversion123/1
  HipMedulla_3L/10(MotorVoltage) -> Data Type Conversion116/1
  HipMedulla_3L/11(LogicVoltage) -> Data Type Conversion118/1
  HipMedulla_3L/12(Thermistor0) -> Data Type Conversion117/1
  HipMedulla_3L/13(Thermistor1) -> Data Type Conversion115/1
  HipMedulla_3L/14(Thermistor2) -> Data Type Conversion158/1
  HipMedulla_3L/15(AmpMeasuredCurrent) -> Data Type Conversion126/1
  Mux1/1 -> EncodeSwitches/1(Switches)
  Mux15/1 -> Ticks/1
  CalibrationParameters/1 -> calibrate/1(CalibrationParams)
  Process Orientation Matrix and Ang Rates/3(IMU_data) -> IMU/1
  Ground/1 -> Data Type Conversion154/1, Data Type Conversion152/1, Data Type Conversion161/1, Data Type Conversion162/1
  Data Type Conversion8/1 -> [ErrorFlags_1L]
  Data Type Conversion9/1 -> [IncEncoder_1L]
  Data Type Conversion10/1 -> [LegEncoderTimestamp_1L]
  Data Type Conversion11/1 -> [MotorEncoderTimestamp_1L]
  Data Type Conversion12/1 -> [IncEncoderTimestamp_1L]
  Data Type Conversion13/1 -> [MotorVoltage_1L]
  Data Type Conversion14/1 -> [LogicVoltage_1L]
  Data Type Conversion15/1 -> [Thermistor0_1L]
  Data Type Conversion16/1 -> [Thermistor1_1L]
  Data Type Conversion17/1 -> [Thermistor2_1L]
  Data Type Conversion18/1 -> [Thermistor3_1L]
  Data Type Conversion19/1 -> [Thermistor4_1L]
  Data Type Conversion20/1 -> [Thermistor5_1L]
  Data Type Conversion21/1 -> [Amp1MeasuredCurrent_1L]
  Data Type Conversion22/1 -> [Amp2MeasuredCurrent_1L]
  Data Type Conversion23/1 -> [KneeForce1_1L]
  Data Type Conversion24/1 -> [KneeForce2_1L]
  [Thermistor0_1R] -> Mux7/1
  [Thermistor1_1R] -> Mux7/2
  [Thermistor2_1R] -> Mux7/3
  [Thermistor3_1R] -> Mux7/4
  [Thermistor4_1R] -> Mux7/5
  [Thermistor5_1R] -> Mux7/6
  [Thermistor0_2R] -> Mux7/7
  [Thermistor1_2R] -> Mux7/8
  [Thermistor2_2R] -> Mux7/9
  [Thermistor3_2R] -> Mux7/10
  [Thermistor4_2R] -> Mux7/11
  [Thermistor5_2R] -> Mux7/12
  [Thermistor0_3R] -> Mux7/13
  [Thermistor1_3R] -> Mux7/14
  [Thermistor2_3R] -> Mux7/15
  [Thermistor0_1L] -> Mux7/16
  [Thermistor1_1L] -> Mux7/17
  [Thermistor2_1L] -> Mux7/18
  [Thermistor3_1L] -> Mux7/19
  [Thermistor4_1L] -> Mux7/20
  [Thermistor5_1L] -> Mux7/21
  [Thermistor0_2L] -> Mux7/22
  [Thermistor1_2L] -> Mux7/23
  [Thermistor2_2L] -> Mux7/24
  [Thermistor3_2L] -> Mux7/25
  [Thermistor4_2L] -> Mux7/26
  [Thermistor5_2L] -> Mux7/27
  [Thermistor0_3L] -> Mux7/28
  [Thermistor1_3L] -> Mux7/29
  [Thermistor2_3L] -> Mux7/30
  Mux7/1 -> ConvertThermistors/1(adc_value)
  [MotorVoltage_1R] -> Mux2/1
  [MotorVoltage_2R] -> Mux2/2
  [MotorVoltage_3R] -> Mux2/3
  [MotorVoltage_1L] -> Mux2/4
  [MotorVoltage_2L] -> Mux2/5
  [MotorVoltage_3L] -> Mux2/6
  [LogicVoltage_1R] -> Mux3/1
  [LogicVoltage_2R] -> Mux3/2
  [LogicVoltage_3R] -> Mux3/3
  [LogicVoltage_1L] -> Mux3/4
  [LogicVoltage_2L] -> Mux3/5
  [LogicVoltage_3L] -> Mux3/6
  [Amp1MeasuredCurrent_1R] -> Mux4/1
  [Amp2MeasuredCurrent_1R] -> Mux4/2
  [Amp1MeasuredCurrent_2R] -> Mux4/3
  [Amp2MeasuredCurrent_2R] -> Mux4/4
  [AmpMeasuredCurrent_3R] -> Mux4/5
  [Amp1MeasuredCurrent_1L] -> Mux4/6
  [Amp2MeasuredCurrent_1L] -> Mux4/7
  [Amp1MeasuredCurrent_2L] -> Mux4/8
  [Amp2MeasuredCurrent_2L] -> Mux4/9
  [AmpMeasuredCurrent_3L] -> Mux4/10
  [State_1R] -> Mux5/1
  [State_2R] -> Mux5/2
  [State_3R] -> Mux5/3
  [State_1L] -> Mux5/4
  [State_2L] -> Mux5/5
  [State_3L] -> Mux5/6
  [ErrorFlags_1R] -> Mux6/1
  [ErrorFlags_2R] -> Mux6/2
  [ErrorFlags_3R] -> Mux6/3
  [ErrorFlags_1L] -> Mux6/4
  [ErrorFlags_2L] -> Mux6/5
  [ErrorFlags_3L] -> Mux6/6
  [ID_1R] -> Mux8/1
  [Counter_1R] -> Mux8/2
  [IncEncoder_1R] -> Mux8/3
  [LegEncoderTimestamp_1R] -> Mux8/4
  [MotorEncoderTimestamp_1R] -> Mux8/5
  [IncEncoderTimestamp_1R] -> Mux8/6
  [KneeForce1_1R] -> Mux8/7
  [KneeForce2_1R] -> Mux8/8
  [ID_2R] -> Mux8/9
  [Counter_2R] -> Mux8/10
  [IncEncoder_2R] -> Mux8/11
  [LegEncoderTimestamp_2R] -> Mux8/12
  [MotorEncoderTimestamp_2R] -> Mux8/13
  [IncEncoderTimestamp_2R] -> Mux8/14
  [KneeForce1_2R] -> Mux8/15
  [KneeForce2_2R] -> Mux8/16
  [ID_3R] -> Mux8/17
  [Counter_3R] -> Mux8/18
  [IncEncoder_3R] -> Mux8/19
  [HipEncoderTimestamp_3R] -> Mux8/20
  [IncEncoderTimestamp_3R] -> Mux8/21
  [ID_1L] -> Mux8/22
  [Counter_1L] -> Mux8/23
  [IncEncoder_1L] -> Mux8/24
  [LegEncoderTimestamp_1L] -> Mux8/25
  [MotorEncoderTimestamp_1L] -> Mux8/26
  [IncEncoderTimestamp_1L] -> Mux8/27
  [KneeForce1_1L] -> Mux8/28
  [KneeForce2_1L] -> Mux8/29
  [ID_2L] -> Mux8/30
  [Counter_2L] -> Mux8/31
  [IncEncoder_2L] -> Mux8/32
  [LegEncoderTimestamp_2L] -> Mux8/33
  [MotorEncoderTimestamp_2L] -> Mux8/34
  [IncEncoderTimestamp_2L] -> Mux8/35
  [KneeForce1_2L] -> Mux8/36
  [KneeForce2_2L] -> Mux8/37
  [ID_3L] -> Mux8/38
  [Counter_3L] -> Mux8/39
  [IncEncoder_3L] -> Mux8/40
  [HipEncoderTimestamp_3L] -> Mux8/41
  [IncEncoderTimestamp_3L] -> Mux8/42
  Mux8/1 -> Terminator3/1
  Data Type Conversion162/1 -> [ID_IMU]
  Data Type Conversion161/1 -> [State_IMU]
  Data Type Conversion152/1 -> [Counter_IMU]
  Data Type Conversion154/1 -> [ErrorFlags_IMU]
  [ID_IMU] -> Mux8/43
  [Counter_IMU] -> Mux8/44
  [ErrorFlags_IMU] -> Mux6/7
  [State_IMU] -> Mux5/7
  Mux2/1 -> ConvertMotorVoltage/1(adc_value)
  Mux3/1 -> ConvertLogicVoltage/1(adc_value)
  Mux4/1 -> ConvertAmpCurrent/1(adc_value)
  Mux5/1 -> MedullaStateVec/1
  Mux6/1 -> ErrorFlagsVec/1
  ConvertMotorVoltage/1(motorVoltage) -> MotorVoltage/1
  ConvertLogicVoltage/1(logicVoltage) -> LogicVoltage/1
  ConvertThermistors/1(temperature) -> Thermistors/1
  ConvertAmpCurrent/1(measuredCurrent) -> AmpMeasuredCurrent/1
  MedullaStateVec/1 -> MedullaState/1  "MedullaState"
  ErrorFlagsVec/1 -> ErrorFlags/1  "ErrorFlags"
  CountersVec/1 -> Terminator5/1
  Mux10/1 -> CountersVec/1
  [Counter_1R] -> Mux10/1
  [Counter_2R] -> Mux10/2
  [Counter_3R] -> Mux10/3
  [Counter_1L] -> Mux10/4
  [Counter_2L] -> Mux10/5
  [Counter_3L] -> Mux10/6
  [Counter_IMU] -> Mux10/7
  Mux17/1 -> [Boom]
  use_imu/1 -> GeneralizedCoordinates/6(UseIMU)
  GeneralizedCoordinates/1(q_clean) -> q/1
  GeneralizedCoordinates/2(dq_clean) -> dq/1
  GeneralizedCoordinates/3(BoomAndIMU) -> BoomAndIMU/1
  Process Orientation Matrix and Ang Rates/2(IMU_Rates) -> [IMU_Rates]
  Data Type Conversion144/1 -> Mux16/8
  Data Type Conversion145/1 -> Mux16/7
  Data Type Conversion131/1 -> Mux16/6
  Data Type Conversion133/1 -> Mux16/5
  Data Type Conversion138/1 -> Mux16/4
  Data Type Conversion132/1 -> Mux16/3
  Data Type Conversion142/1 -> Mux16/2
  Data Type Conversion143/1 -> Mux16/1
  Data Type Conversion139/1 -> Mux17/3
  Data Type Conversion140/1 -> Mux17/2
  Data Type Conversion141/1 -> Mux17/1
  BoomMedulla/3(PitchEncoder) -> Data Type Conversion139/1
  BoomMedulla/4(ID) -> Data Type Conversion143/1
  BoomMedulla/5(State) -> Data Type Conversion142/1
  BoomMedulla/6(Counter) -> Data Type Conversion132/1
  BoomMedulla/7(ErrorFlags) -> Data Type Conversion138/1
  BoomMedulla/8(Z_EncoderTimestamp) -> Data Type Conversion133/1
  BoomMedulla/9(OSU_X_EncoderTimestamp) -> Data Type Conversion131/1
  BoomMedulla/10(PitchEncoderTimestamp) -> Data Type Conversion145/1
  BoomMedulla/11(LogicVoltage) -> Data Type Conversion144/1
  Mux16/1 -> Terminator4/1
  Counter/1 -> [MedullaCounter]
  [MedullaCounter] -> LegMedulla_1L/2(MedullaCounter)
  [MedullaCounter] -> HipMedulla_3L/2(MedullaCounter)
  [MedullaCounter] -> HipMedulla_3R/2(MedullaCounter)
  [MedullaCounter] -> LegMedulla_2R/2(MedullaCounter)
  [MedullaCounter] -> LegMedulla_1R/2(MedullaCounter)
  [MedullaCounter] -> LegMedulla_2L/2(MedullaCounter)
  [MedullaCommand] -> LegMedulla_1R/1(MedullaCmd)
  [MedullaCommand] -> LegMedulla_2R/1(MedullaCmd)
  [MedullaCommand] -> LegMedulla_2L/1(MedullaCmd)
  [MedullaCommand] -> LegMedulla_1L/1(MedullaCmd)
  [MedullaCommand] -> HipMedulla_3R/1(MedullaCmd)
  [MedullaCommand] -> HipMedulla_3L/1(MedullaCmd)
  [MedullaCommand] -> BoomMedulla/1(MedullaCmd)
  [MedullaCounter] -> BoomMedulla/2(MedullaCounter)
  [MotorCommand_1L] -> LegMedulla_1L/3(MotorCmd)
  [MotorCommand_2L] -> LegMedulla_2L/3(MotorCmd)
  [MotorCommand_1R] -> LegMedulla_1R/3(MotorCmd)
  [MotorCommand_2R] -> LegMedulla_2R/3(MotorCmd)
  [MotorCommand_3R] -> HipMedulla_3R/3(MotorCmd)
  Demux1/6 -> [MotorCommand_3L]
  [MotorCommand_3L] -> HipMedulla_3L/3(MotorCmd)
  Demux1/1 -> [MotorCommand_1L]
  Demux1/2 -> [MotorCommand_2L]
  Demux1/3 -> [MotorCommand_1R]
  Demux1/4 -> [MotorCommand_2R]
  Demux1/5 -> [MotorCommand_3R]
  Data Type Conversion157/1 -> [LimitSwitch_3R]
  Data Type Conversion112/1 -> [LimitSwitch_3L]
  [LimitSwitch_1R] -> Mux1/1
  [LimitSwitch_2R] -> Mux1/2
  [LimitSwitch_3R] -> Mux1/3
  [LimitSwitch_1L] -> Mux1/4
  [LimitSwitch_2L] -> Mux1/5
  [LimitSwitch_3L] -> Mux1/6
  [ToeSensor_1R] -> Mux11/1
  [ToeSensor_2R] -> Mux11/2
  [ToeSensor_1L] -> Mux11/3
  [ToeSensor_2L] -> Mux11/4
  Data Type Conversion76/1 -> [LimitSwitch_2R]
  Data Type Conversion75/1 -> [ToeSensor_2R]
  Data Type Conversion51/1 -> [ToeSensor_1R]
  Data Type Conversion52/1 -> [LimitSwitch_1R]
  Data Type Conversion27/1 -> [ToeSensor_2L]
  Data Type Conversion28/1 -> [LimitSwitch_2L]
  Data Type Conversion2/1 -> [ToeSensor_1L]
  Data Type Conversion4/1 -> [LimitSwitch_1L]
  Process Orientation Matrix and Ang Rates/1(IMU_Angles) -> [IMU_Angles]
  Data Type Conversion3/1 -> [LegEncoder_1L]
  Data Type Conversion1/1 -> [MotorEncoder_1L]
  Data Type Conversion25/1 -> [LegEncoder_2L]
  Data Type Conversion26/1 -> [MotorEncoder_2L]
  Data Type Conversion49/1 -> [LegEncoder_1R]
  Data Type Conversion50/1 -> [MotorEncoder_1R]
  Data Type Conversion73/1 -> [LegEncoder_2R]
  Data Type Conversion74/1 -> [MotorEncoder_2R]
  [IncEncoder_1R] -> Mux12/1
  [IncEncoder_2R] -> Mux12/2
  [IncEncoder_3R] -> Mux12/5
  [IncEncoder_1L] -> Mux12/3
  [IncEncoder_2L] -> Mux12/4
  [IncEncoder_3L] -> Mux12/6
  [LegEncoder_1R] -> Mux14/1
  [LegEncoder_2R] -> Mux14/2
  [LegEncoder_1L] -> Mux14/3
  [LegEncoder_2L] -> Mux14/4
  Mux12/1 -> [IncEncoders]
  Mux14/1 -> [AbsEncoders]
  [AbsEncoders] -> Mux15/1
  [IncEncoders] -> Mux15/2
  [Boom] -> Mux15/3
  IMU Command/1 -> Terminator8/1
  [AbsEncoders] -> calibrate/2(AbsEncoders)
  calibrate/3(Rollover) -> Unit Delay/1
  Unit Delay/1 -> calibrate/6(RolloverIn)
  [MotorEncoder_1R] -> Mux14/5
  [MotorEncoder_2R] -> Mux14/6
  [MotorEncoder_1L] -> Mux14/7
  [MotorEncoder_2L] -> Mux14/8
  [HipEncoder_3R] -> Mux14/9
  [HipEncoder_3L] -> Mux14/10
  [Reset] -> calibrate/5(Reset)
  Reset/1(Reset) -> [Reset]
  ResetDAQ/1 -> Reset/1(ResetIn)
  Unit Delay1/1 -> calibrate/4(IncEncodersPrev)
  [IncEncoders] -> Mux9/1
  [Boom] -> Mux9/2
  Mux9/1 -> calibrate/3(IncEncoders), Unit Delay1/1
  Unit Delay2/1 -> calibrate/7(IncCalTickIn)
  calibrate/4(IncCalTick) -> Unit Delay2/1
  [IMU_Angles] -> IMUFilters/1
  [Reset] -> EncoderFilters/4
  [Reset] -> IMUFilters/4
  UseIMURates/1 -> IMUFilters/6
  [IMU_Rates] -> IMUFilters/5
  calibrate/1(AbsAngle) -> Vector Concatenate/1
  calibrate/2(IncAngle) -> Vector Concatenate/2
  Vector Concatenate/1 -> EncoderFilters/1, EncodersDirty/1
  EncoderAngleLimits/1 -> EncoderFilters/2
  EncoderThreshold/1 -> EncoderFilters/3
  IMUThreshold/1 -> IMUFilters/3
  IMUAngleLimits/1 -> IMUFilters/2
  IMUTorsoOffset/1 -> GeneralizedCoordinates/7(IMUTorsoOffset)
  GearOffset/1 -> GeneralizedCoordinates/8(GearOffset)
  [Reset] -> GeneralizedCoordinates/9(Reset)
  UseMotorIncEncoders/1 -> GeneralizedCoordinates/5(UseMotorIncEncoders)
  IMUFilters/2 -> GeneralizedCoordinates/4(IMUVelocities)
  IMUFilters/1 -> GeneralizedCoordinates/3(IMUAngles)
  EncoderFilters/2 -> GeneralizedCoordinates/2(EncoderVelocities)
  EncoderFilters/1 -> GeneralizedCoordinates/1(EncoderAngles), EncodersClean/1
  EncoderFilters/3 -> [ErrorCountEncoders]
  IMUFilters/3 -> [ErrorCountIMU]
  Mux18/1 -> ErrorCounts/1
  [ErrorCountEncoders] -> Mux18/1
  [ErrorCountIMU] -> Mux18/2
